simulink library "LumAerospaceBlockset_Utilities"  (R2021a)
settings: Solver=ode45  StartTime=0.0  StopTime=10.0  RelTol=1e-3  EnableMultiTasking=on
undefined symbols (not defined in the file): magnitude
libraries: $bdroot x8, LumMiscBlockset x2
settings Model: Creator=Christopher  LastModifiedBy=chris
settings SolverCC: AlgebraicLoopSolver=TrustRegion
settings DataIOCC: LimitDataPoints=on  SaveFormat=Array  ReturnWorkspaceOutputs=off
settings OptimizationCC: LifeSpan=inf
settings DebuggingCC: SolverPrmCheckMsg=warning  SFUnexpectedBacktrackingDiag=warning  SFNoUnconditionalDefaultTransitionDiag=warning  SFExecutionAtInitializationDiag=none  SFMachineParentedDataDiag=warning  ArithmeticOperatorsInVariantConditions=warning
settings HardwareCC: ProdBitPerPointer=32  ProdBitPerSizeT=32  ProdBitPerPtrDiffT=32  ProdLargestAtomicFloat=None  ProdIntDivRoundTo=Undefined  ProdEndianess=Unspecified  ProdWordSize=32  ProdHWDeviceType=32-bit Generic
settings ModelReferenceCC: PropagateSignalLabelsOutOfModel=off
settings SFSimCC: SimUseLocalCustomCode=off  CustomCodeUndefinedFunction=UseInterfaceOnly
settings RTWCC: RTWUseLocalCustomCode=off
settings CodeAppCC: StateflowObjectComments=on
settings GRTTargetCC: TargetLangStandard=C89/C90 (ANSI)
settings ConfigComp: CovMetricSettings=dw  CovSaveCumulativeToWorkspaceVar=on  CovSaveSingleToWorkspaceVar=on  CovExternalEMLEnable=off  CovSFcnEnable=off

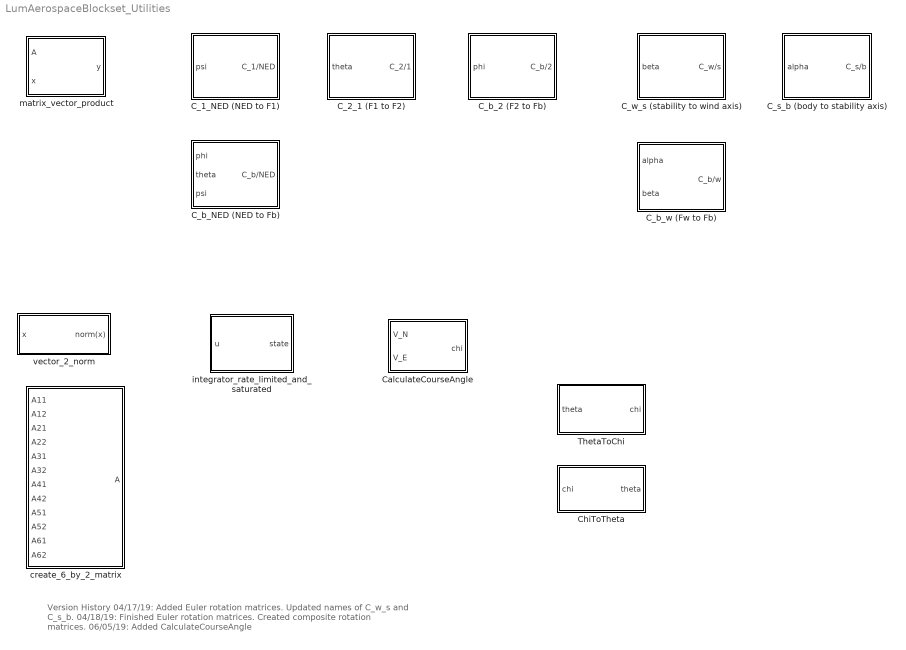
== system LumAerospaceBlockset_Utilities ==
  note: Version History
      | 04/17/19: Added Euler rotation matrices.  Updated names of C_w_s and C_s_b.
      | 04/18/19: Finished Euler rotation matrices.  Created composite rotation matrices.
      | 06/05/19: Added CalculateCourseAngle
  C_1_NED (NED to F1) : Subsystem
      mask help:
      | This rotation matrix can be used to transform a vector expressed in the North/East/Down frame (F_NED) to a vector expressed it in the F_1 frame.
      |
      | Consider two frames, F_NED and F_1.  F_1 is obtained by rotating F_NED about the z axis through angle psi.  This block computes the rotation matrix which can be applied to a vector expressed in F_NED to obtain the vector expressed in F_1.
      |
      | Example
      |
      |    vector_NED = ...
      |    vector_1 = C_1_NED(psi)*vector_NED
      |
      | This matrix is given by
      |
      |          [ cos(psi) sin(psi) 0]
      |          [-sin(psi) cos(psi) 0]
      |          [ 0        0        1]
      |
      | INPUT:     -psi:   the rotation angle (rad)
      |
      | OUTPUT:    -C_1/NED:     3x3 rotation matrix
      |
      | See also RotationMatrices.C_1_NED
      |
      | Created by Christopher Lum
      | lum@uw.edu
  C_2_1 (F1 to F2) : Subsystem
      mask help:
      | This rotation matrix can be used to transform a vector expressed in the F_1 frame to a vector expressed it in the F_2 frame.
      |
      | Consider two frames, F_1 and F_2.  F_2 is obtained by rotating F_1 about the y axis through angle theta.
      |
      | This method computes the rotation matrix which can be applied to a vector expressed in F_1 to obtain the vector expressed in F_2.
      |
      | Example
      |
      |    vector_1 = ...
      |    vector_2 = C_2_1(theta)*vector_1;
      |
      | This matrix is given by
      |
      |          [cos(theta) 0 -sin(theta)]
      |          [0          1  0         ]
      |          [sin(theta) 0  cos(theta)]
      |
      | INPUT:     -theta:   the rotation angle (rad)
      |
      | OUTPUT:    -C_2/1:     3x3 rotation matrix
      |
      | See also RotationMatrices.C_2_1
      |
      | Created by Christopher Lum
      | lum@uw.edu
  C_b_2 (F2 to Fb) : Subsystem
      mask help:
      | This rotation matrix can be used to transform a vector expressed in the F_2 frame to a vector expressed it in the F_b frame.
      |
      | Consider two frames, F_2 and F_b.  F_b is obtained by rotating F_2 about the x axis through angle phi.
      |
      | This computes the rotation matrix which can be applied to a vector expressed in F_2 to obtain the vector expressed in F_b.
      |
      | Example
      |
      |    vector_2 = ...
      |    vector_b = RotationMatrices.C_b_2(phi)*vector_2;
      |
      | This matrix is given by
      |
      |          [1  0        0       ]
      |          [0  cos(phi) sin(phi)]
      |          [0 -sin(phi) cos(phi)]
      |
      | INPUT:     -phi:   the rotation angle (a UWAngle object)
      |
      | OUTPUT:    -C_b/2:     3x3 rotation matrix
      |
      | See also RotationMatrices.C_b_2
      |
      | Created by Christopher Lum
      | lum@uw.edu
  C_b_NED (NED to Fb) : Subsystem
      mask help:
      | This rotation matrix can be used to transform a vector expressed in the F_NED frame to a vector expressed it in the F_b frame.
      |
      | Example
      |
      |    vector_NED = ...
      |    vector_b = C_b_NED(phi, theta, psi)*vector_NED
      |
      | INPUT:     	phi:	x-rotation angle (rad)
      | 	theta:	y-rotation angle (rad)
      | 	psi:   	z-rotation angle (rad)
      |
      | OUTPUT:    -C_b/NED:     3x3 rotation matrix
      |
      | See also RotationMatrices.C_b_NED
      |
      | Created by Christopher Lum
      | lum@uw.edu
  C_b_w (Fw to Fb) : Subsystem
      mask help:
      | This rotation matrix can be used to transform a vector expressed in the F_w (wind) frame to a vector expressed it in the F_b (body) frame.
      |
      |    V_b = C_b_w(alpha, beta)*V_w
      |
      | INPUT:     	alpha:	angle of attack (rad)
      | 	beta:	angle of sideslip (rad)
      |
      | OUTPUT:    -C_b/w:     3x3 rotation matrix
      |
      | See also RotationMatrices.C_b_w_lite
      |
      | Created by Christopher Lum
      | lum@uw.edu
  C_s_b (body to stability axis) : Subsystem
      mask help:
      | Compute the rotation matrix from body to stability axis
      |
      | C_s/b = [ cos(alpha) 0  sin(alpha);
      |           0          1  0
      |          -sin(alpha) 0  cos(alpha)]
      |
      | INPUT:  alpha: angle of attack
      |
      | OUTPUT: C_s/b: direction cosine matrix to transform from body to stability axis.
  C_w_s (stability to wind axis) : Subsystem
      mask help:
      | Compute the rotation matrix from stability to wind axis
      |
      | C_w/s = [ cos(beta) sin(beta) 0;
      |          -sin(beta) cos(beta) 0
      |           0         0         1]
      |
      | INPUT:  beta: side slip angle
      |
      | OUTPUT: C_w/s: direction cosine matrix to transform from stability to wind axis.
  CalculateCourseAngle : Subsystem
      mask help:
      | Calculate the course angle (chie) given the north velocity (V_N) and east velocity (V_E).
      |
      | A heading of chi = 0 implies a course of directly north.
      |
      | The units of V_N and V_E must be teh same.  chi is restricted to the range of [0, 2*pi).
      |
      | INPUTS:
      | -V_N: North velocity
      | -V_E: East velocity
      |
      | OUTPUTS:
      | -chi: course angle in range of [0, 2*pi) (radians)
      |
      | Created by Christopher Lum
      | lum@uw.edu
  ChiToTheta : Subsystem
      mask help:
      | See 'ThetaToChi' as this block is simly the reverse of that operation.
      |
      | Created by Christopher Lum
      | lum@uw.edu
  ThetaToChi : Subsystem
      mask help:
      | Convert and angle from theta to chi.
      |
      | theta = 0 implies pointing directly East with positive theta measured counter-clockwise
      | chi = 0 implies pointing directly North with positive chi measured clockwise.
      |
      | theta is typically used when dealing with simple planar vehicles whereas chi is typically used with navigation (course or bearing angles).
      |
      | INPUTS:
      | -theta: angle from Eastward (radians)
      |
      | OUTPUTS
      | -chi: angel from Northward (radians, restricted to output range of [0,2*pi) )
      |
      | Created by Christopher Lum
      | lum@uw.edu
  create_6_by_2_matrix : Subsystem
      mask help:
      | Create a 6-by-2 matrix from 12 input values.  Each input coresponds to an element of hte matrix.
      |
      | For example, the input labeld A21 is the entry in the second row and first column of the matrix.
      |
      | INPUT:  -A11:   row 1, col 1 entry
      |         -A12:   row 1, col 2 entry
      |         -A21:   row 2, col 1 entry
      |         .
      |         .
      |         .
      |         -A62:   row 6, col 2 entry
      |
      | OUTPUT: -A: 6-by-2 matrix
      |
      | VALIDATION: -unit test
  integrator_rate_limited_and_saturated : Subsystem  mask{x0=0, rate_gain=1, x_max=10, x_min=-10}
      mask prompts: x0 "Initial state (unit)"; rate_gain "Maximum state change rate (unit/s)"; x_max "Maximum state (unit)"; x_min "Minimum state (unit)"
      mask help:
      | Models an integrator where the state is both saturated and rate limited.
      |
      | Saturated implies that the state of the integrator is limited to a minimum value of 'Minimum state' and a maximum value of 'Maximum state'.
      |
      | Rate limited implies that the state of the integrator cannot change faster than the 'Maximum state change rate'.
      |
      | If the input 'u' is at +1, the state of the integrator will change by the 'Maximum state change rate'.  Conversely, if the input 'u' is -1, the state of the integrator will change by -'Maximum state change rate'.  Values of 'u' outside the range [-1,1] are saturated to [-1,1].
      |
      | INPUT:  -u: input in range [-1,1]
      |
      | OUTPUT: -state: state of the integrator
      |
      | VALIDATION: -unit test
  matrix_vector_product : Subsystem
      mask help:
      | Performs matrix and vector multiplication
      |
      |     y = A*x
      |
      | INPUT:  A: matrix to multiply
      |         x: vector to multiply
      |
      | OUTPUT: y: product of A*x
  vector_2_norm : Subsystem
      mask help:
      | Compute the 2-norm of a 3 dimensional vector
      |
      |     y = norm(x) = sqrt(x(1)^2 + x(2)^2 + x(3)^2)
      |
      | INPUT:  x:  3x1 vector
      |
      | OUTPUT: norm(x):    2-norm of x
      |
      | VALIDATION: none

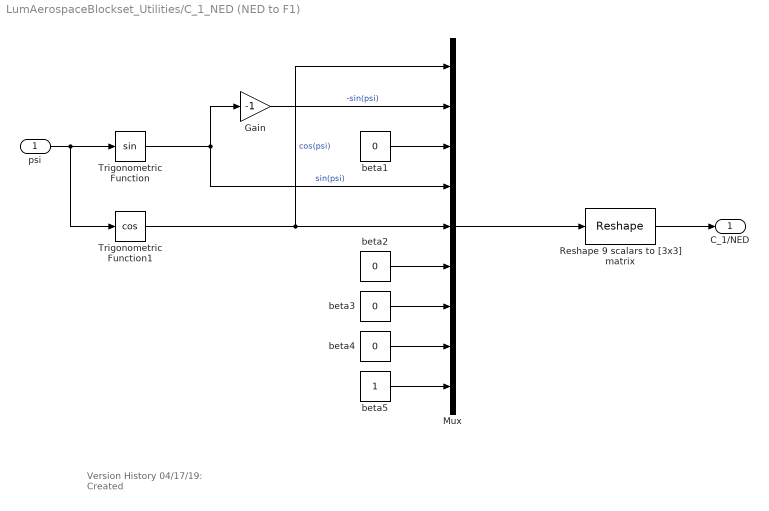
== system LumAerospaceBlockset_Utilities/C_1_NED (NED to F1) ==
  note: Version History
      | 04/17/19: Created
  psi : Inport
  Gain : Gain  Gain=-1
  Mux : Mux  Inputs=9
  Reshape 9 scalars to [3x3] matrix : Reshape  OutputDimensionality=Customize  OutputDimensions=[3,3]
  Trigonometric Function : Trigonometry
  Trigonometric Function1 : Trigonometry  Operator=cos
  beta{1..4} (4 alike) : Constant  Value=0
  beta5 : Constant
  C_1/NED : Outport  VectorParamsAs1DForOutWhenUnconnected=off
  wires:
  Gain/1 -> Mux/2  "-sin(psi)"
  beta1/1 -> Mux/3
  Mux/1 -> Reshape 9 scalars to [3x3] matrix/1
  psi/1 -> Trigonometric Function1/1, Trigonometric Function/1
  Trigonometric Function1/1 -> Mux/5, Mux/1  "cos(psi)"
  Reshape 9 scalars to [3x3] matrix/1 -> C_1/NED/1
  Trigonometric Function/1 -> Mux/4, Gain/1  "sin(psi)"
  beta2/1 -> Mux/6
  beta3/1 -> Mux/7
  beta4/1 -> Mux/8
  beta5/1 -> Mux/9

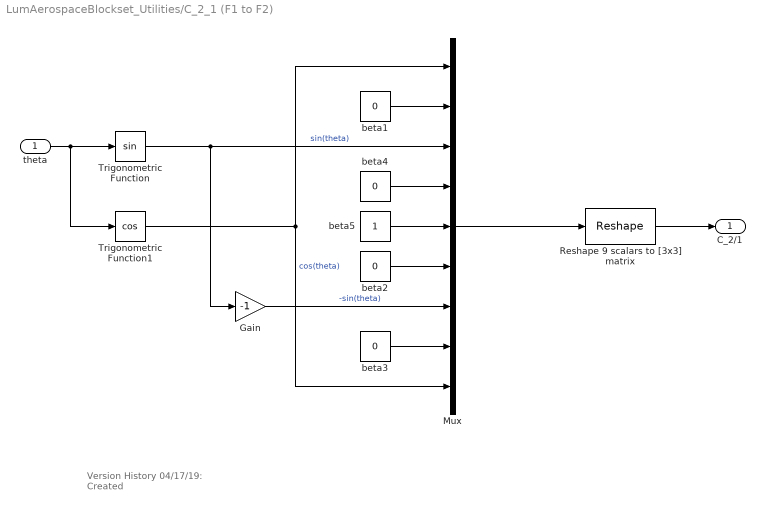
== system LumAerospaceBlockset_Utilities/C_2_1 (F1 to F2) ==
  note: Version History
      | 04/17/19: Created
  theta : Inport
  Gain : Gain  Gain=-1
  Mux : Mux  Inputs=9
  Reshape 9 scalars to [3x3] matrix : Reshape  OutputDimensionality=Customize  OutputDimensions=[3,3]
  Trigonometric Function : Trigonometry
  Trigonometric Function1 : Trigonometry  Operator=cos
  beta{1..4} (4 alike) : Constant  Value=0
  beta5 : Constant
  C_2/1 : Outport  VectorParamsAs1DForOutWhenUnconnected=off
  wires:
  Trigonometric Function/1 -> Mux/3, Gain/1  "sin(theta)"
  Reshape 9 scalars to [3x3] matrix/1 -> C_2/1/1
  Trigonometric Function1/1 -> Mux/9, Mux/1  "cos(theta)"
  theta/1 -> Trigonometric Function/1, Trigonometric Function1/1
  Mux/1 -> Reshape 9 scalars to [3x3] matrix/1
  Gain/1 -> Mux/7  "-sin(theta)"
  beta1/1 -> Mux/2
  beta4/1 -> Mux/4
  beta5/1 -> Mux/5
  beta2/1 -> Mux/6
  beta3/1 -> Mux/8

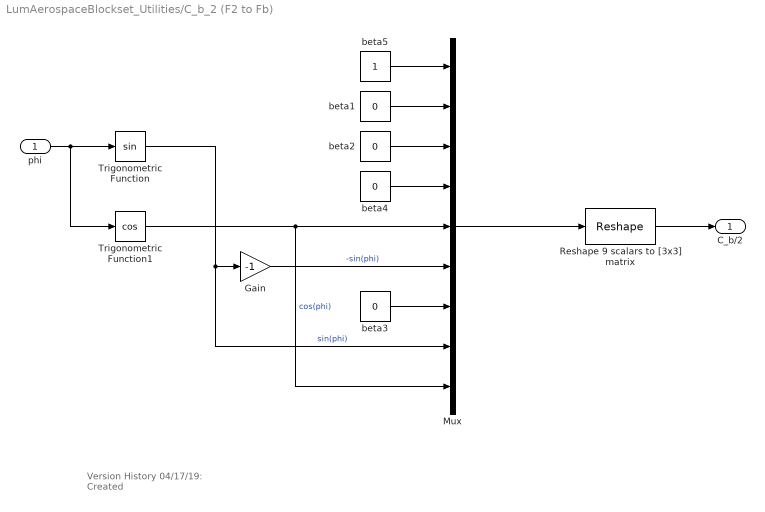
== system LumAerospaceBlockset_Utilities/C_b_2 (F2 to Fb) ==
  note: Version History
      | 04/17/19: Created
  phi : Inport
  Gain : Gain  Gain=-1
  Mux : Mux  Inputs=9
  Reshape 9 scalars to [3x3] matrix : Reshape  OutputDimensionality=Customize  OutputDimensions=[3,3]
  Trigonometric Function : Trigonometry
  Trigonometric Function1 : Trigonometry  Operator=cos
  beta{1..4} (4 alike) : Constant  Value=0
  beta5 : Constant
  C_b/2 : Outport  VectorParamsAs1DForOutWhenUnconnected=off
  wires:
  beta4/1 -> Mux/4
  beta1/1 -> Mux/2
  Gain/1 -> Mux/6  "-sin(phi)"
  Mux/1 -> Reshape 9 scalars to [3x3] matrix/1
  phi/1 -> Trigonometric Function1/1, Trigonometric Function/1
  Trigonometric Function1/1 -> Mux/9, Mux/5  "cos(phi)"
  Reshape 9 scalars to [3x3] matrix/1 -> C_b/2/1
  Trigonometric Function/1 -> Gain/1, Mux/8  "sin(phi)"
  beta5/1 -> Mux/1
  beta2/1 -> Mux/3
  beta3/1 -> Mux/7

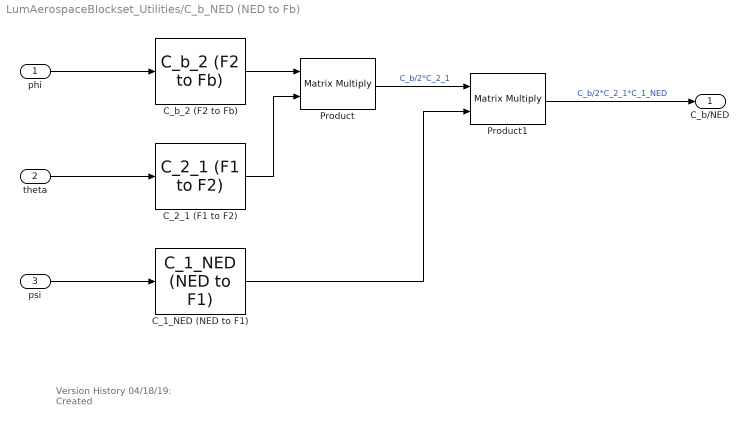
== system LumAerospaceBlockset_Utilities/C_b_NED (NED to Fb) ==
  note: Version History
      | 04/18/19: Created
  phi : Inport
  theta : Inport  Port=2
  psi : Inport  Port=3
  C_1_NED (NED to F1) : $bdroot/C_1_NED (NED to F1)
  C_2_1 (F1 to F2) : $bdroot/C_2_1 (F1 to F2)
  C_b_2 (F2 to Fb) : $bdroot/C_b_2 (F2 to Fb)
  Product : Product  Multiplication=Matrix(*)
  Product1 : Product  Multiplication=Matrix(*)
  C_b/NED : Outport  VectorParamsAs1DForOutWhenUnconnected=off
  wires:
  phi/1 -> C_b_2 (F2 to Fb)/1
  theta/1 -> C_2_1 (F1 to F2)/1
  psi/1 -> C_1_NED (NED to F1)/1
  C_b_2 (F2 to Fb)/1 -> Product/1
  C_2_1 (F1 to F2)/1 -> Product/2
  Product/1 -> Product1/1  "C_b/2*C_2_1"
  C_1_NED (NED to F1)/1 -> Product1/2
  Product1/1 -> C_b/NED/1  "C_b/2*C_2_1*C_1_NED"

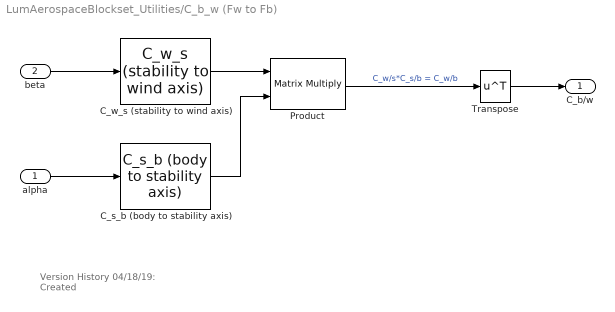
== system LumAerospaceBlockset_Utilities/C_b_w (Fw to Fb) ==
  note: Version History
      | 04/18/19: Created
  alpha : Inport
  beta : Inport  Port=2
  C_s_b (body to stability axis) : $bdroot/C_s_b (body to stability axis)
  C_w_s (stability to wind axis) : $bdroot/C_w_s (stability to wind axis)
  Product : Product  Multiplication=Matrix(*)
  Transpose : Math  Operator=transpose  SignedPower=on  SaturateOnIntegerOverflow=on
  C_b/w : Outport  VectorParamsAs1DForOutWhenUnconnected=off
  wires:
  Product/1 -> Transpose/1  "C_w/s*C_s/b = C_w/b"
  alpha/1 -> C_s_b (body to stability axis)/1
  beta/1 -> C_w_s (stability to wind axis)/1
  C_w_s (stability to wind axis)/1 -> Product/1
  C_s_b (body to stability axis)/1 -> Product/2
  Transpose/1 -> C_b/w/1

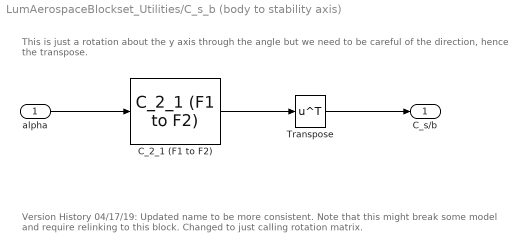
== system LumAerospaceBlockset_Utilities/C_s_b (body to stability axis) ==
  note: Version History
      | 04/17/19: Updated name to be more consistent.  Note that this might break some model and require relinking to this block.  Changed to just calling rotation matrix.
  note: This is just a rotation about the y axis through the angle but we need to be careful of the direction, hence the transpose.
  alpha : Inport
  C_2_1 (F1 to F2) : $bdroot/C_2_1 (F1 to F2)
  Transpose : Math  Operator=transpose  SignedPower=on  SaturateOnIntegerOverflow=on
  C_s/b : Outport  VectorParamsAs1DForOutWhenUnconnected=off
  wires:
  alpha/1 -> C_2_1 (F1 to F2)/1
  C_2_1 (F1 to F2)/1 -> Transpose/1
  Transpose/1 -> C_s/b/1

== system LumAerospaceBlockset_Utilities/C_w_s (stability to wind axis) ==
  note: This is just a rotation about the z axis through the angle so use equivalent rotation matrix block.
  note: Version History
      | 04/17/19: Updated name to be more consistent.  Note that this might break some model and require relinking to this block.  Changed to just call other rotation matrix block.
  beta : Inport
  C_1_NED (NED to F1) : $bdroot/C_1_NED (NED to F1)
  C_w/s : Outport  VectorParamsAs1DForOutWhenUnconnected=off
  wires:
  beta/1 -> C_1_NED (NED to F1)/1
  C_1_NED (NED to F1)/1 -> C_w/s/1

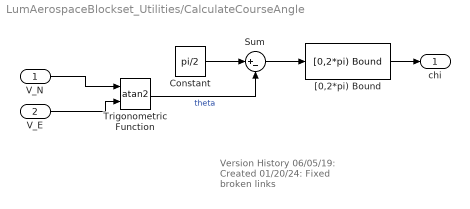
== system LumAerospaceBlockset_Utilities/CalculateCourseAngle ==
  note: Version History
      | 06/05/19: Created
      | 01/20/24: Fixed broken links
  V_N : Inport
  V_E : Inport  Port=2
  Constant : Constant  Value=pi/2
  Sum : Sum  Inputs=|+-
  Trigonometric Function : Trigonometry  Operator=atan2
  "[0,2*pi) Bound" : LumMiscBlockset/[0,2*pi) Bound  Description=|
      | Version History  
      |                  
      | 05/??/05: Created
  chi : Outport  VectorParamsAs1DForOutWhenUnconnected=off
  wires:
  V_N/1 -> Trigonometric Function/1
  V_E/1 -> Trigonometric Function/2
  "[0,2*pi) Bound"/1 -> chi/1
  Trigonometric Function/1 -> Sum/2  "theta"
  Constant/1 -> Sum/1
  Sum/1 -> "[0,2*pi) Bound"/1

== system LumAerospaceBlockset_Utilities/ChiToTheta ==
  note: The conversion is the same so simply use the 'ThetaToChi' block
  chi : Inport
  ThetaToChi : $bdroot/ThetaToChi
  theta : Outport  VectorParamsAs1DForOutWhenUnconnected=off
  wires:
  chi/1 -> ThetaToChi/1
  ThetaToChi/1 -> theta/1

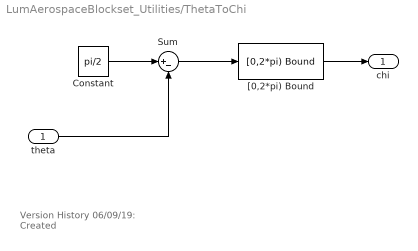
== system LumAerospaceBlockset_Utilities/ThetaToChi ==
  note: Version History
      | 06/09/19: Created
  theta : Inport
  Constant : Constant  Value=pi/2
  Sum : Sum  Inputs=|+-
  "[0,2*pi) Bound" : LumMiscBlockset/[0,2*pi) Bound  Description=|
      | Version History  
      |                  
      | 05/??/05: Created
  chi : Outport  VectorParamsAs1DForOutWhenUnconnected=off
  wires:
  "[0,2*pi) Bound"/1 -> chi/1
  Constant/1 -> Sum/1
  theta/1 -> Sum/2
  Sum/1 -> "[0,2*pi) Bound"/1

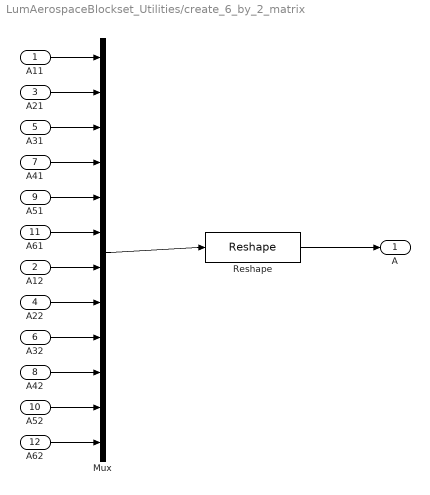
== system LumAerospaceBlockset_Utilities/create_6_by_2_matrix ==
  A11 : Inport
  A12 : Inport  Port=2
  A21 : Inport  Port=3
  A22 : Inport  Port=4
  A31 : Inport  Port=5
  A32 : Inport  Port=6
  A41 : Inport  Port=7
  A42 : Inport  Port=8
  A51 : Inport  Port=9
  A52 : Inport  Port=10
  A61 : Inport  Port=11
  A62 : Inport  Port=12
  Mux : Mux  Inputs=12
  Reshape : Reshape  OutputDimensionality=Customize  OutputDimensions=[6,2]
  A : Outport  VectorParamsAs1DForOutWhenUnconnected=off
  wires:
  Reshape/1 -> A/1
  Mux/1 -> Reshape/1
  A62/1 -> Mux/12
  A52/1 -> Mux/11
  A42/1 -> Mux/10
  A32/1 -> Mux/9
  A22/1 -> Mux/8
  A12/1 -> Mux/7
  A61/1 -> Mux/6
  A51/1 -> Mux/5
  A41/1 -> Mux/4
  A31/1 -> Mux/3
  A21/1 -> Mux/2
  A11/1 -> Mux/1

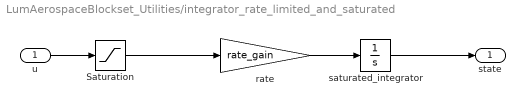
== system LumAerospaceBlockset_Utilities/integrator_rate_limited_and_saturated ==
  u : Inport
  Saturation : Saturate  UpperLimit=1  LowerLimit=-1
  rate : Gain  Gain=rate_gain  SaturateOnIntegerOverflow=on  OutDataTypeStr=Inherit: Same as input  ParamDataTypeStr=Inherit: Same as input
  saturated_integrator : Integrator  InitialCondition=x0  LimitOutput=on  UpperSaturationLimit=x_max  LowerSaturationLimit=x_min
  state : Outport  VectorParamsAs1DForOutWhenUnconnected=off
  wires:
  saturated_integrator/1 -> state/1
  rate/1 -> saturated_integrator/1
  Saturation/1 -> rate/1
  u/1 -> Saturation/1

== system LumAerospaceBlockset_Utilities/matrix_vector_product ==
  A : Inport
  x : Inport  Port=2
  Product : Product  Multiplication=Matrix(*)  RndMeth=Zero
  y : Outport  VectorParamsAs1DForOutWhenUnconnected=off
  wires:
  Product/1 -> y/1
  A/1 -> Product/1
  x/1 -> Product/2

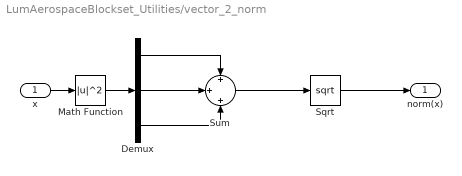
== system LumAerospaceBlockset_Utilities/vector_2_norm ==
  x : Inport
  Demux : Demux  Outputs=3
  Math Function : Math  Operator=magnitude^2  SignedPower=on  SaturateOnIntegerOverflow=on
  Sqrt : Sqrt  SaturateOnIntegerOverflow=on
  Sum : Sum  Inputs=+|+|+
  norm(x) : Outport  VectorParamsAs1DForOutWhenUnconnected=off
  wires:
  Sqrt/1 -> norm(x)/1
  Sum/1 -> Sqrt/1
  Demux/3 -> Sum/3
  Demux/2 -> Sum/2
  Demux/1 -> Sum/1
  Math Function/1 -> Demux/1
  x/1 -> Math Function/1
